simulink model "Proyecto_Global_AyCD_Ultimo2"  (R2017b)
settings: Solver=FixedStepAuto  StartTime=0.0  StopTime=inf  FixedStep=0.01  RelTol=1e-3  EnableMultiTasking=on
values from neighbouring files (symbols this model uses):
  AhMax = 1    [datosAyCD.m]
  AtMax = 1    [datosAyCD.m]
  Ba_b = zeros(1,60)    [PD_balanceo_CARGA_GainScheduling.m]
  Ba_h = Mh*n_h*Wpos_h    [PID_izaje_CARGA.m]
  Ba_t = Mt*n_t*Wpos_t    [PID_traslacion_CARRO.m]
  bContenedor = 2.5    [datosAyCD.m]
  bh = bhEq*rh^2/Rd^2    (= 28800)    [datosAyCD.m]
  bt = btEq*rt^2/Rw^2    (= 27000)    [datosAyCD.m]
  bw = 30000    [datosAyCD.m]
  cantidadCarrilesBarco = 9+1    (= 10)    [datosAyCD.m]
  g = 9.80665    [datosAyCD.m]
  hContenedor = 2.5    [datosAyCD.m]
  hLimInf = -17.5-2    (= -19.5)    [datosAyCD.m]
  hLimSup = 40+2    (= 42)    [datosAyCD.m]
  Kd = zeros(1,60)    [PD_balanceo_CARGA_AutoTunning.m]
  Kp = zeros(1,60)    [PD_balanceo_CARGA_AutoTunning.m]
  Ksa_b = zeros(1,60)    [PD_balanceo_CARGA_GainScheduling.m]
  Ksa_h = Mh*n_h*Wpos_h^2    [PID_izaje_CARGA.m]
  Ksa_t = Mt*n_t*Wpos_t^2    [PID_traslacion_CARRO.m]
  Ksia_h = Mh*Wpos_h^3    [PID_izaje_CARGA.m]
  Ksia_t = Mt*Wpos_t^3    [PID_traslacion_CARRO.m]
  Kw = 1800000    [datosAyCD.m]
  l1 = zeros(1,60)    [PD_balanceo_CARGA_AutoTunning.m]
  Mh = (Jd+Jmh*rh^2) / (Rd^2)    (= 48014.2222222)    [datosAyCD.m]
  mlMax = mlMin+48000    (= 65000)    [datosAyCD.m]
  mlVacio = 15000    [datosAyCD.m]
  Mt = mc + (Jw+Jmt*rt^2) / (Rw^2)    (= 59008)    [datosAyCD.m]
  nRand = [14 17 20 22 20 17 14 8 8 8]    [datosAyCD.m]
  Rd = 0.75    [datosAyCD.m]
  rh = 30    [datosAyCD.m]
  rt = 15    [datosAyCD.m]
  Rw = 0.5    [datosAyCD.m]
  Tf = zeros(1,60)    [PD_balanceo_CARGA_AutoTunning.m]
  tLimDer = 50+2    (= 52)    [datosAyCD.m]
  tLimIzq = -30-2    (= -32)    [datosAyCD.m]
  VhMaxC = 1.5    [datosAyCD.m]
  VhMaxV = 3    [datosAyCD.m]
  xCarrilBarco = zeros(1,cantidadCarrilesBarco)    [datosAyCD.m]
  xCarrilMuelle = [-30,-25,-20,-15,-10,-5]    [datosAyCD.m]
  yCarrilBarcoPar = zeros(1,cantidadCarrilesBarco)    [datosAyCD.m]
  ySB = 15    [datosAyCD.m]
  yt0 = 45    [datosAyCD.m]
undefined symbols (not defined in the file or in its folder): lh
libraries: simulink x5
(part 2 of 2)

== stateflow chart Proyecto_Global_AyCD_Ultimo2/Nivel 0 ==
  state NORMAL
    entry: Vh0=0; Vt0=0;
    state SITUACION_NORMAL
      entry:
      Alarma=0;
    state EMERGENCIA_FIN_CARRERA
      entry:
      Alarma=1;
    state EMERGENCIA_PULSADOR
      entry:
      Alarma=1;
    state EMERGENCIA_SOBREVELOCIDAD
      entry:
      Alarma=1;
    (default) -> SITUACION_NORMAL
    SITUACION_NORMAL -> EMERGENCIA_FIN_CARRERA [order 1] : [(fcL==1)||(fcR==1)]
    SITUACION_NORMAL -> EMERGENCIA_FIN_CARRERA [order 5] : [(fcU==1)||(fcD==1)]
    SITUACION_NORMAL -> EMERGENCIA_PULSADOR [order 3] : [Emergencia==1]
    SITUACION_NORMAL -> EMERGENCIA_SOBREVELOCIDAD [order 4] : [ (Dlh>VhMax*1.1) || (Dlh<-VhMax*1.1) ]
    SITUACION_NORMAL -> EMERGENCIA_SOBREVELOCIDAD [order 2] : [ (Dxt>VtMax*1.1)  ||  (Dxt<-VtMax*1.1) ]
  state EMERGENCIA
    entry:
    Vt0=0; Vh0=0;
    state MANUAL_EMERGENCIA
      during:
      calculaVt0_emergencia();
      calculaVh0_emergencia();
    state APAGAR_ALARMA
      entry:
      Vt0=0; Vh0=0; Alarma=0;
    (default) -> MANUAL_EMERGENCIA
    MANUAL_EMERGENCIA -> APAGAR_ALARMA : [Reiniciar==1]
  (default) -> NORMAL
  NORMAL -> EMERGENCIA : [Alarma==1]
  EMERGENCIA -> NORMAL : [Alarma==0]
  data: fcL input; fcR input; fcU input; fcD input; Vh0 output double; Vt0 output double; Dxt input; Dlh input; Reiniciar input; Emergencia input; VtMax input; VhMax input; Alarma output double
  function calculaVt0_emergencia:
    | function calculaVt0_emergencia
    | 
    | if((fcR==0) ||(fcL==0)) 
    |      Vt0 = VtMax/3;
    | else
    |      Vt0 = 0;
    | end
  function calculaVh0_emergencia:
    | function calculaVh0_emergencia %Descenso de ida
    | 
    | if( (fcD==0) || (fcU==0))
    |     Vh0 = VhMax/3;
    | else
    |     Vh0 = 0;
    | end
    | 
    | if ( (fcR==0)&&(fcL==0)&&(fcU==0)&&(fcD==0) )
    |     Revision = 0;
    | else 
    |     Revision = 1;
    | end
